simulink model "w3p1"  (R2020b)
settings: Solver=VariableStepAuto  StartTime=0.0  StopTime=10.0  RelTol=1e-3
settings Model: Creator=family  LastModifiedBy=family

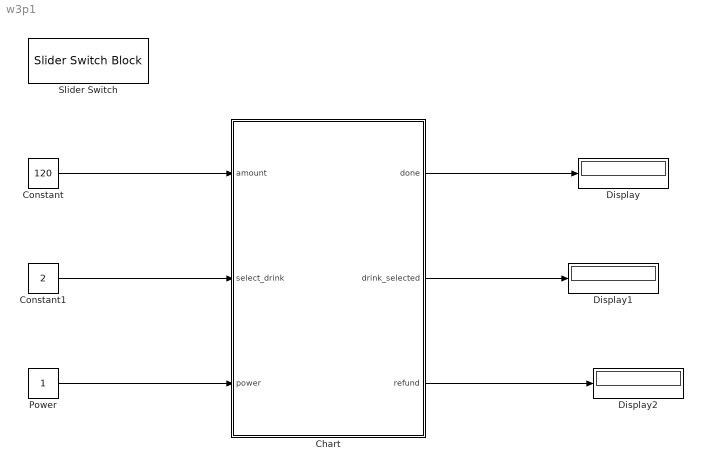
== system w3p1 ==
  Chart : Stateflow chart  TreatAsAtomicUnit=on
  Constant : Constant  Value=120
  Constant1 : Constant  Value=2
  Display : Display
  Display1 : Display
  Display2 : Display
  Power : Constant
  Slider Switch : SliderSwitchBlock
      settings: Values={{'Off', 'On'}, [0 1]}
  wires:
  Chart/3(refund) -> Display2/1
  Chart/1(done) -> Display/1
  Constant1/1 -> Chart/2(select_drink)
  Constant/1 -> Chart/1(amount)
  Power/1 -> Chart/3(power)
  Chart/2(drink_selected) -> Display1/1

== stateflow chart w3p1/Chart ==
  state On
    state Idle
    state Wait
    state Wait_for_selection
    state Refund
    state Dispensing
    Idle -> Wait : [amount>0&&done==0]
    (default) -> Idle
    Wait -> Wait [order 3] : [amount<drink_cost]
    Wait -> Refund [order 1] : after(5,sec)
    Refund -> Idle : [done==1]{refund=amount-drink_cost;}
    Wait -> Wait_for_selection [order 2] : [amount>=drink_cost]{done=0;}
    Wait_for_selection -> Refund [order 1] : after(5,sec)
    Wait_for_selection -> Dispensing [order 2] : [select_drink>0]{drink_selected=select_drink;}
    Dispensing -> Refund : after(2,sec){done=1;}
  state Off
  Off -> On : [power==1]
  (default) -> Off
  On -> Off : [power==0]
  data: drink_cost local =10; done output =0; amount input; select_drink input; drink_selected output; refund output; power input
